simulink model "test_YAN_fusion"  (R2020b)
settings: Solver=ode1  StartTime=t0  StopTime=tf  FixedStep=0.004  RelTol=1e-3  EnableMultiTasking=on
values from neighbouring files (symbols this model uses):
  IMU = IN_SENSOR.IMU1    [run_simulation.m]
undefined symbols (not defined in the file or in its folder): accel_x, accel_y, accel_z, airspeed, airspeed1, airspeed2, airspeed3, airspeed_calibrate, airspeed_indicate, airspeed_true, alt_baro, baro1, baro2, BESTPOS, delta_height, delta_lat, delta_lon, dynamic_pressure, EAS2TAS_Algo, flag, Flag, glv, gyro_x, gyro_y, gyro_z, hAcc, headAcc, height, IMU1, IMU1_Control, IMU2, IMU3, IMU4, laserDown1, laserDown2, Lat, Lon, mag1, mag2, mag_x, mag_y, mag_z, nChange, numSv, pDop, radar1, radarLongDown1, radarLongForward1, range, Range, sAcc, SNR, static_pressure, status, strength, temperature, time, ublox1, um482, vAcc ... (+3)
(part 2 of 3)

== system test_YAN_fusion/SOURCE lookup table/laserDown1 ==
  time : Inport
  1-D Lookup Table1 : Lookup_n-D  NumberOfTableDimensions=1  BreakpointsForDimension1=IN_SENSOR.laserDown1.time(1:end-20)  Table=IN_SENSOR.laserDown1.range(1:end-20)  InterpMethod=Flat  ExtrapMethod=Clip  InternalRulePriority=Speed  RndMeth=Simplest  InputSameDT=on
  1-D Lookup Table2 : Lookup_n-D  NumberOfTableDimensions=1  BreakpointsForDimension1=IN_SENSOR.laserDown1.time(1:end-20)  Table=IN_SENSOR.laserDown1.flag(1:end-20)  InterpMethod=Flat  ExtrapMethod=Clip  InternalRulePriority=Speed  RndMeth=Simplest  InputSameDT=on
  1-D Lookup Table3 : Lookup_n-D  NumberOfTableDimensions=1  BreakpointsForDimension1=IN_SENSOR.laserDown1.time(1:end-20)  Table=IN_SENSOR.laserDown1.strength(1:end-20)  InterpMethod=Flat  ExtrapMethod=Clip  InternalRulePriority=Speed  RndMeth=Simplest  InputSameDT=on
  1-D Lookup Table4 : Lookup_n-D  NumberOfTableDimensions=1  BreakpointsForDimension1=IN_SENSOR.laserDown1.time(1:end-20)  Table=IN_SENSOR.laserDown1.nChange(1:end-20)  InterpMethod=Flat  ExtrapMethod=Clip  InternalRulePriority=Speed  RndMeth=Simplest  InputSameDT=on
  1-D Lookup Table9 : Lookup_n-D  NumberOfTableDimensions=1  BreakpointsForDimension1=IN_SENSOR.laserDown1.time(1:end-20)  Table=IN_SENSOR.laserDown1.time(1:end-20)  InterpMethod=Flat  ExtrapMethod=Clip  InternalRulePriority=Speed  RndMeth=Simplest  InputSameDT=on
  Bus Assignment : BusAssignment  AssignedSignals=time,range,flag,strength,nChange
  Constant : Constant  Value=0  OutDataTypeStr=Bus: BUS_LASERR_DOWN
  Data Type Conversion{,1..4} (5 alike) : DataTypeConversion
  Gain{1..3,8} (4 alike) : Gain
  Outport : Outport
  wires:
  time/1 -> 1-D Lookup Table1/1, 1-D Lookup Table9/1, 1-D Lookup Table2/1, 1-D Lookup Table4/1, 1-D Lookup Table3/1
  1-D Lookup Table3/1 -> Data Type Conversion3/1
  Data Type Conversion3/1 -> Gain3/1
  Data Type Conversion2/1 -> Gain2/1
  1-D Lookup Table2/1 -> Data Type Conversion2/1
  1-D Lookup Table1/1 -> Data Type Conversion1/1
  Data Type Conversion1/1 -> Gain1/1
  Data Type Conversion/1 -> Gain8/1
  1-D Lookup Table9/1 -> Data Type Conversion/1
  Gain3/1 -> Bus Assignment/5  "strength"
  Gain2/1 -> Bus Assignment/4  "flag"
  Gain8/1 -> Bus Assignment/2  "time"
  Gain1/1 -> Bus Assignment/3  "range"
  Constant/1 -> Bus Assignment/1
  Bus Assignment/1 -> Outport/1
  1-D Lookup Table4/1 -> Data Type Conversion4/1
  Data Type Conversion4/1 -> Bus Assignment/6  "nChange"

== system test_YAN_fusion/SOURCE lookup table/laserDown2 ==
  time : Inport
  1-D Lookup Table1 : Lookup_n-D  NumberOfTableDimensions=1  BreakpointsForDimension1=IN_SENSOR.laserDown2.time(1:end-20)  Table=IN_SENSOR.laserDown2.range(1:end-20)  InterpMethod=Flat  ExtrapMethod=Clip  InternalRulePriority=Speed  RndMeth=Simplest  InputSameDT=on
  1-D Lookup Table2 : Lookup_n-D  NumberOfTableDimensions=1  BreakpointsForDimension1=IN_SENSOR.laserDown2.time(1:end-20)  Table=IN_SENSOR.laserDown2.flag(1:end-20)  InterpMethod=Flat  ExtrapMethod=Clip  InternalRulePriority=Speed  RndMeth=Simplest  InputSameDT=on
  1-D Lookup Table3 : Lookup_n-D  NumberOfTableDimensions=1  BreakpointsForDimension1=IN_SENSOR.laserDown2.time(1:end-20)  Table=IN_SENSOR.laserDown2.strength(1:end-20)  InterpMethod=Flat  ExtrapMethod=Clip  InternalRulePriority=Speed  RndMeth=Simplest  InputSameDT=on
  1-D Lookup Table4 : Lookup_n-D  NumberOfTableDimensions=1  BreakpointsForDimension1=IN_SENSOR.laserDown2.time(1:end-20)  Table=IN_SENSOR.laserDown2.nChange(1:end-20)  InterpMethod=Flat  ExtrapMethod=Clip  InternalRulePriority=Speed  RndMeth=Simplest  InputSameDT=on
  1-D Lookup Table9 : Lookup_n-D  NumberOfTableDimensions=1  BreakpointsForDimension1=IN_SENSOR.laserDown2.time(1:end-20)  Table=IN_SENSOR.laserDown2.time(1:end-20)  InterpMethod=Flat  ExtrapMethod=Clip  InternalRulePriority=Speed  RndMeth=Simplest  InputSameDT=on
  Bus Assignment : BusAssignment  AssignedSignals=time,range,flag,strength,nChange
  Constant : Constant  Value=0  OutDataTypeStr=Bus: BUS_LASERR_DOWN
  Data Type Conversion{,1..4} (5 alike) : DataTypeConversion
  Gain{1..3,8} (4 alike) : Gain
  Outport : Outport
  wires:
  time/1 -> 1-D Lookup Table1/1, 1-D Lookup Table9/1, 1-D Lookup Table2/1, 1-D Lookup Table4/1, 1-D Lookup Table3/1
  1-D Lookup Table3/1 -> Data Type Conversion3/1
  Data Type Conversion3/1 -> Gain3/1
  Data Type Conversion2/1 -> Gain2/1
  1-D Lookup Table2/1 -> Data Type Conversion2/1
  1-D Lookup Table1/1 -> Data Type Conversion1/1
  Data Type Conversion1/1 -> Gain1/1
  Data Type Conversion/1 -> Gain8/1
  1-D Lookup Table9/1 -> Data Type Conversion/1
  Gain3/1 -> Bus Assignment/5  "strength"
  Gain2/1 -> Bus Assignment/4  "flag"
  Gain8/1 -> Bus Assignment/2  "time"
  Gain1/1 -> Bus Assignment/3  "range"
  Constant/1 -> Bus Assignment/1
  Data Type Conversion4/1 -> Bus Assignment/6  "nChange"
  1-D Lookup Table4/1 -> Data Type Conversion4/1
  Bus Assignment/1 -> Outport/1

== system test_YAN_fusion/SOURCE lookup table/mag1 ==
  time : Inport
  1-D Lookup Table1 : Lookup_n-D  NumberOfTableDimensions=1  BreakpointsForDimension1=IN_SENSOR.mag1.time(1:end-20)  Table=IN_SENSOR.mag1.mag_x(1:end-20)  InterpMethod=Flat  ExtrapMethod=Clip  InternalRulePriority=Speed  RndMeth=Simplest  InputSameDT=on
  1-D Lookup Table2 : Lookup_n-D  NumberOfTableDimensions=1  BreakpointsForDimension1=IN_SENSOR.mag1.time(1:end-20)  Table=IN_SENSOR.mag1.mag_y(1:end-20)  InterpMethod=Flat  ExtrapMethod=Clip  InternalRulePriority=Speed  RndMeth=Simplest  InputSameDT=on
  1-D Lookup Table3 : Lookup_n-D  NumberOfTableDimensions=1  BreakpointsForDimension1=IN_SENSOR.mag1.time(1:end-20)  Table=IN_SENSOR.mag1.mag_z(1:end-20)  InterpMethod=Flat  ExtrapMethod=Clip  InternalRulePriority=Speed  RndMeth=Simplest  InputSameDT=on
  1-D Lookup Table4 : Lookup_n-D  NumberOfTableDimensions=1  BreakpointsForDimension1=IN_SENSOR.mag1.time(1:end-20)  Table=IN_SENSOR.mag1.nChange(1:end-20)  InterpMethod=Flat  ExtrapMethod=Clip  InternalRulePriority=Speed  RndMeth=Simplest  InputSameDT=on
  1-D Lookup Table9 : Lookup_n-D  NumberOfTableDimensions=1  BreakpointsForDimension1=IN_SENSOR.mag1.time(1:end-20)  Table=IN_SENSOR.mag1.time(1:end-20)  InterpMethod=Flat  ExtrapMethod=Clip  InternalRulePriority=Speed  RndMeth=Simplest  InputSameDT=on
  Bus Assignment : BusAssignment  AssignedSignals=time,mag_x,mag_y,mag_z,nChange
  Constant : Constant  Value=0  OutDataTypeStr=Bus: BUS_MAG
  Data Type Conversion{,1..4} (5 alike) : DataTypeConversion
  Gain{1..4} (4 alike) : Gain
  Outport : Outport
  wires:
  Gain3/1 -> Bus Assignment/2  "time"
  Gain1/1 -> Bus Assignment/3  "mag_x"
  Gain4/1 -> Bus Assignment/5  "mag_z"
  Gain2/1 -> Bus Assignment/4  "mag_y"
  Data Type Conversion/1 -> Gain3/1
  1-D Lookup Table9/1 -> Data Type Conversion/1
  1-D Lookup Table1/1 -> Data Type Conversion1/1
  Data Type Conversion1/1 -> Gain1/1
  Data Type Conversion2/1 -> Gain2/1
  1-D Lookup Table2/1 -> Data Type Conversion2/1
  1-D Lookup Table3/1 -> Data Type Conversion3/1
  Data Type Conversion3/1 -> Gain4/1
  time/1 -> 1-D Lookup Table4/1, 1-D Lookup Table3/1, 1-D Lookup Table2/1, 1-D Lookup Table1/1, 1-D Lookup Table9/1
  Constant/1 -> Bus Assignment/1
  Bus Assignment/1 -> Outport/1
  1-D Lookup Table4/1 -> Data Type Conversion4/1
  Data Type Conversion4/1 -> Bus Assignment/6  "nChange"

== system test_YAN_fusion/SOURCE lookup table/mag2 ==
  time : Inport
  1-D Lookup Table1 : Lookup_n-D  NumberOfTableDimensions=1  BreakpointsForDimension1=IN_SENSOR.mag2.time(1:end-20)  Table=IN_SENSOR.mag2.mag_x(1:end-20)  InterpMethod=Flat  ExtrapMethod=Clip  InternalRulePriority=Speed  RndMeth=Simplest  InputSameDT=on
  1-D Lookup Table2 : Lookup_n-D  NumberOfTableDimensions=1  BreakpointsForDimension1=IN_SENSOR.mag2.time(1:end-20)  Table=IN_SENSOR.mag2.mag_y(1:end-20)  InterpMethod=Flat  ExtrapMethod=Clip  InternalRulePriority=Speed  RndMeth=Simplest  InputSameDT=on
  1-D Lookup Table3 : Lookup_n-D  NumberOfTableDimensions=1  BreakpointsForDimension1=IN_SENSOR.mag2.time(1:end-20)  Table=IN_SENSOR.mag2.mag_z(1:end-20)  InterpMethod=Flat  ExtrapMethod=Clip  InternalRulePriority=Speed  RndMeth=Simplest  InputSameDT=on
  1-D Lookup Table4 : Lookup_n-D  NumberOfTableDimensions=1  BreakpointsForDimension1=IN_SENSOR.mag2.time(1:end-20)  Table=IN_SENSOR.mag2.nChange(1:end-20)  InterpMethod=Flat  ExtrapMethod=Clip  InternalRulePriority=Speed  RndMeth=Simplest  InputSameDT=on
  1-D Lookup Table9 : Lookup_n-D  NumberOfTableDimensions=1  BreakpointsForDimension1=IN_SENSOR.mag2.time(1:end-20)  Table=IN_SENSOR.mag2.time(1:end-20)  InterpMethod=Flat  ExtrapMethod=Clip  InternalRulePriority=Speed  RndMeth=Simplest  InputSameDT=on
  Bus Assignment : BusAssignment  AssignedSignals=time,mag_x,mag_y,mag_z,nChange
  Constant : Constant  Value=0  OutDataTypeStr=Bus: BUS_MAG
  Data Type Conversion{,1..4} (5 alike) : DataTypeConversion
  Gain{1..4} (4 alike) : Gain
  Outport : Outport
  wires:
  Data Type Conversion4/1 -> Bus Assignment/6  "nChange"
  1-D Lookup Table4/1 -> Data Type Conversion4/1
  Bus Assignment/1 -> Outport/1
  Constant/1 -> Bus Assignment/1
  time/1 -> 1-D Lookup Table9/1, 1-D Lookup Table1/1, 1-D Lookup Table2/1, 1-D Lookup Table3/1, 1-D Lookup Table4/1
  Data Type Conversion3/1 -> Gain4/1
  1-D Lookup Table3/1 -> Data Type Conversion3/1
  1-D Lookup Table2/1 -> Data Type Conversion2/1
  Data Type Conversion2/1 -> Gain2/1
  Data Type Conversion1/1 -> Gain1/1
  1-D Lookup Table1/1 -> Data Type Conversion1/1
  1-D Lookup Table9/1 -> Data Type Conversion/1
  Data Type Conversion/1 -> Gain3/1
  Gain2/1 -> Bus Assignment/4  "mag_y"
  Gain4/1 -> Bus Assignment/5  "mag_z"
  Gain1/1 -> Bus Assignment/3  "mag_x"
  Gain3/1 -> Bus Assignment/2  "time"

== system test_YAN_fusion/SOURCE lookup table/radar1 ==
  time : Inport
  1-D Lookup Table1 : Lookup_n-D  NumberOfTableDimensions=1  BreakpointsForDimension1=IN_SENSOR.radar1.time(1:end-20)  Table=IN_SENSOR.radar1.SNR(1:end-20)  InterpMethod=Flat  ExtrapMethod=Clip  InternalRulePriority=Speed  RndMeth=Simplest  InputSameDT=on
  1-D Lookup Table2 : Lookup_n-D  NumberOfTableDimensions=1  BreakpointsForDimension1=IN_SENSOR.radar1.time(1:end-20)  Table=IN_SENSOR.radar1.Flag(1:end-20)  InterpMethod=Flat  ExtrapMethod=Clip  InternalRulePriority=Speed  RndMeth=Simplest  InputSameDT=on
  1-D Lookup Table3 : Lookup_n-D  NumberOfTableDimensions=1  BreakpointsForDimension1=IN_SENSOR.radar1.time(1:end-20)  Table=IN_SENSOR.radar1.Range(1:end-20)  InterpMethod=Flat  ExtrapMethod=Clip  InternalRulePriority=Speed  RndMeth=Simplest  InputSameDT=on
  1-D Lookup Table4 : Lookup_n-D  NumberOfTableDimensions=1  BreakpointsForDimension1=IN_SENSOR.radar1.time(1:end-20)  Table=IN_SENSOR.radar1.nChange(1:end-20)  InterpMethod=Flat  ExtrapMethod=Clip  InternalRulePriority=Speed  RndMeth=Simplest  InputSameDT=on
  1-D Lookup Table9 : Lookup_n-D  NumberOfTableDimensions=1  BreakpointsForDimension1=IN_SENSOR.radar1.time(1:end-20)  Table=IN_SENSOR.radar1.time(1:end-20)  InterpMethod=Flat  ExtrapMethod=Clip  InternalRulePriority=Speed  RndMeth=Simplest  InputSameDT=on
  Bus Assignment : BusAssignment  AssignedSignals=time,SNR,Flag,Range,nChange
  Constant : Constant  Value=0  OutDataTypeStr=Bus: BUS_RADAR
  Data Type Conversion{,1..4} (5 alike) : DataTypeConversion
  Gain{1..4} (4 alike) : Gain
  Outport : Outport
  wires:
  Gain3/1 -> Bus Assignment/2  "time"
  Gain1/1 -> Bus Assignment/3  "SNR"
  Gain4/1 -> Bus Assignment/5  "Range"
  Gain2/1 -> Bus Assignment/4  "Flag"
  1-D Lookup Table9/1 -> Data Type Conversion/1
  Data Type Conversion/1 -> Gain3/1
  Data Type Conversion1/1 -> Gain1/1
  1-D Lookup Table1/1 -> Data Type Conversion1/1
  1-D Lookup Table2/1 -> Data Type Conversion2/1
  Data Type Conversion2/1 -> Gain2/1
  Data Type Conversion3/1 -> Gain4/1
  1-D Lookup Table3/1 -> Data Type Conversion3/1
  time/1 -> 1-D Lookup Table4/1, 1-D Lookup Table3/1, 1-D Lookup Table2/1, 1-D Lookup Table1/1, 1-D Lookup Table9/1
  Constant/1 -> Bus Assignment/1
  Bus Assignment/1 -> Outport/1
  1-D Lookup Table4/1 -> Data Type Conversion4/1
  Data Type Conversion4/1 -> Bus Assignment/6  "nChange"

== system test_YAN_fusion/SOURCE lookup table/radarLongDown1 ==
  time : Inport
  1-D Lookup Table1 : Lookup_n-D  NumberOfTableDimensions=1  BreakpointsForDimension1=IN_SENSOR.radarLongDown1.time(1:end-20)  Table=IN_SENSOR.radarLongDown1.range(1:end-20)  InterpMethod=Flat  ExtrapMethod=Clip  InternalRulePriority=Speed  RndMeth=Simplest  InputSameDT=on
  1-D Lookup Table2 : Lookup_n-D  NumberOfTableDimensions=1  BreakpointsForDimension1=IN_SENSOR.radarLongDown1.time(1:end-20)  Table=IN_SENSOR.radarLongDown1.flag(1:end-20)  InterpMethod=Flat  ExtrapMethod=Clip  InternalRulePriority=Speed  RndMeth=Simplest  InputSameDT=on
  1-D Lookup Table3 : Lookup_n-D  NumberOfTableDimensions=1  BreakpointsForDimension1=IN_SENSOR.radarLongDown1.time(1:end-20)  Table=IN_SENSOR.radarLongDown1.strength(1:end-20)  InterpMethod=Flat  ExtrapMethod=Clip  InternalRulePriority=Speed  RndMeth=Simplest  InputSameDT=on
  1-D Lookup Table4 : Lookup_n-D  NumberOfTableDimensions=1  BreakpointsForDimension1=IN_SENSOR.radarLongDown1.time(1:end-20)  Table=IN_SENSOR.radarLongDown1.nChange(1:end-20)  InterpMethod=Flat  ExtrapMethod=Clip  InternalRulePriority=Speed  RndMeth=Simplest  InputSameDT=on
  1-D Lookup Table9 : Lookup_n-D  NumberOfTableDimensions=1  BreakpointsForDimension1=IN_SENSOR.radarLongDown1.time(1:end-20)  Table=IN_SENSOR.radarLongDown1.time(1:end-20)  InterpMethod=Flat  ExtrapMethod=Clip  InternalRulePriority=Speed  RndMeth=Simplest  InputSameDT=on
  Bus Assignment : BusAssignment  AssignedSignals=time,range,flag,strength,nChange
  Constant : Constant  Value=0  OutDataTypeStr=Bus: BUS_RADAR_LONG
  Data Type Conversion{,1..4} (5 alike) : DataTypeConversion
  Gain{1..3,8} (4 alike) : Gain
  Outport : Outport
  wires:
  Gain1/1 -> Bus Assignment/3  "range"
  Gain8/1 -> Bus Assignment/2  "time"
  Gain2/1 -> Bus Assignment/4  "flag"
  Gain3/1 -> Bus Assignment/5  "strength"
  1-D Lookup Table9/1 -> Data Type Conversion/1
  Data Type Conversion/1 -> Gain8/1
  Data Type Conversion1/1 -> Gain1/1
  1-D Lookup Table1/1 -> Data Type Conversion1/1
  1-D Lookup Table2/1 -> Data Type Conversion2/1
  Data Type Conversion2/1 -> Gain2/1
  Data Type Conversion3/1 -> Gain3/1
  1-D Lookup Table3/1 -> Data Type Conversion3/1
  time/1 -> 1-D Lookup Table4/1, 1-D Lookup Table3/1, 1-D Lookup Table9/1, 1-D Lookup Table1/1, 1-D Lookup Table2/1
  Constant/1 -> Bus Assignment/1
  Data Type Conversion4/1 -> Bus Assignment/6  "nChange"
  1-D Lookup Table4/1 -> Data Type Conversion4/1
  Bus Assignment/1 -> Outport/1

== system test_YAN_fusion/SOURCE lookup table/radarLongForward1 ==
  time : Inport
  1-D Lookup Table1 : Lookup_n-D  NumberOfTableDimensions=1  BreakpointsForDimension1=IN_SENSOR.radarLongForward1.time(1:end-20)  Table=IN_SENSOR.radarLongForward1.range(1:end-20)  InterpMethod=Flat  ExtrapMethod=Clip  InternalRulePriority=Speed  RndMeth=Simplest  InputSameDT=on
  1-D Lookup Table2 : Lookup_n-D  NumberOfTableDimensions=1  BreakpointsForDimension1=IN_SENSOR.radarLongForward1.time(1:end-20)  Table=IN_SENSOR.radarLongForward1.flag(1:end-20)  InterpMethod=Flat  ExtrapMethod=Clip  InternalRulePriority=Speed  RndMeth=Simplest  InputSameDT=on
  1-D Lookup Table3 : Lookup_n-D  NumberOfTableDimensions=1  BreakpointsForDimension1=IN_SENSOR.radarLongForward1.time(1:end-20)  Table=IN_SENSOR.radarLongForward1.strength(1:end-20)  InterpMethod=Flat  ExtrapMethod=Clip  InternalRulePriority=Speed  RndMeth=Simplest  InputSameDT=on
  1-D Lookup Table4 : Lookup_n-D  NumberOfTableDimensions=1  BreakpointsForDimension1=IN_SENSOR.radarLongForward1.time(1:end-20)  Table=IN_SENSOR.radarLongForward1.nChange(1:end-20)  InterpMethod=Flat  ExtrapMethod=Clip  InternalRulePriority=Speed  RndMeth=Simplest  InputSameDT=on
  1-D Lookup Table9 : Lookup_n-D  NumberOfTableDimensions=1  BreakpointsForDimension1=IN_SENSOR.radarLongForward1.time(1:end-20)  Table=IN_SENSOR.radarLongForward1.time(1:end-20)  InterpMethod=Flat  ExtrapMethod=Clip  InternalRulePriority=Speed  RndMeth=Simplest  InputSameDT=on
  Bus Assignment : BusAssignment  AssignedSignals=time,range,flag,strength,nChange
  Constant : Constant  Value=0  OutDataTypeStr=Bus: BUS_RADAR_LONG
  Data Type Conversion{,1..4} (5 alike) : DataTypeConversion
  Gain{1..3,8} (4 alike) : Gain
  Outport : Outport
  wires:
  time/1 -> 1-D Lookup Table1/1, 1-D Lookup Table9/1, 1-D Lookup Table2/1, 1-D Lookup Table4/1, 1-D Lookup Table3/1
  1-D Lookup Table3/1 -> Data Type Conversion3/1
  Data Type Conversion3/1 -> Gain3/1
  Data Type Conversion2/1 -> Gain2/1
  1-D Lookup Table2/1 -> Data Type Conversion2/1
  1-D Lookup Table1/1 -> Data Type Conversion1/1
  Data Type Conversion1/1 -> Gain1/1
  Data Type Conversion/1 -> Gain8/1
  1-D Lookup Table9/1 -> Data Type Conversion/1
  Gain3/1 -> Bus Assignment/5  "strength"
  Gain2/1 -> Bus Assignment/4  "flag"
  Gain8/1 -> Bus Assignment/2  "time"
  Gain1/1 -> Bus Assignment/3  "range"
  Constant/1 -> Bus Assignment/1
  Bus Assignment/1 -> Outport/1
  1-D Lookup Table4/1 -> Data Type Conversion4/1
  Data Type Conversion4/1 -> Bus Assignment/6  "nChange"

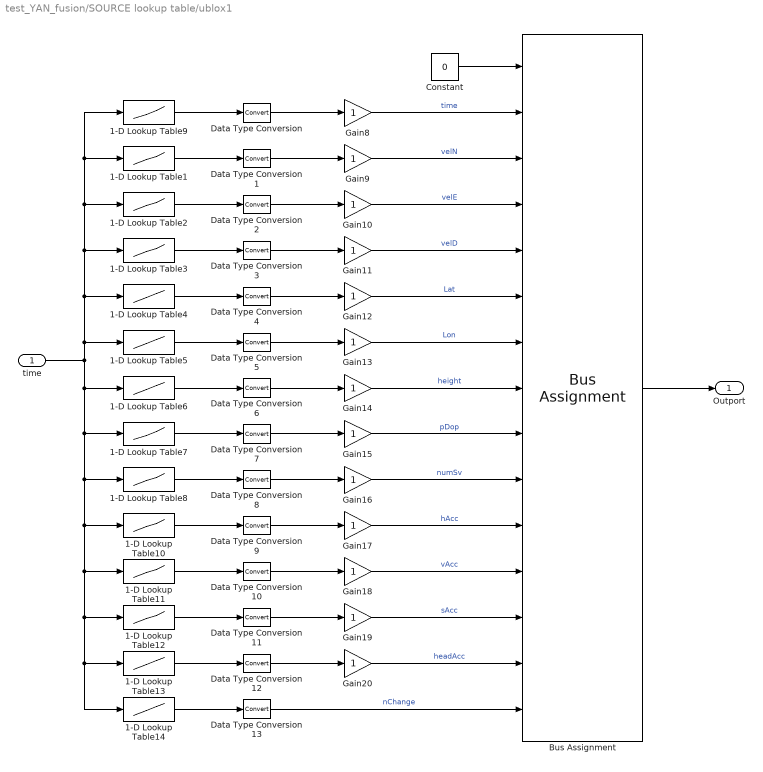
== system test_YAN_fusion/SOURCE lookup table/ublox1 ==
  time : Inport
  1-D Lookup Table1 : Lookup_n-D  NumberOfTableDimensions=1  BreakpointsForDimension1=IN_SENSOR.ublox1.time(1:end-20)  Table=IN_SENSOR.ublox1.velN(1:end-20)  InterpMethod=Flat  ExtrapMethod=Clip  InternalRulePriority=Speed  RndMeth=Simplest  InputSameDT=on
  1-D Lookup Table10 : Lookup_n-D  NumberOfTableDimensions=1  BreakpointsForDimension1=IN_SENSOR.ublox1.time(1:end-20)  Table=IN_SENSOR.ublox1.hAcc(1:end-20)  InterpMethod=Flat  ExtrapMethod=Clip  InternalRulePriority=Speed  RndMeth=Simplest  InputSameDT=on
  1-D Lookup Table11 : Lookup_n-D  NumberOfTableDimensions=1  BreakpointsForDimension1=IN_SENSOR.ublox1.time(1:end-20)  Table=IN_SENSOR.ublox1.vAcc(1:end-20)  InterpMethod=Flat  ExtrapMethod=Clip  InternalRulePriority=Speed  RndMeth=Simplest  InputSameDT=on
  1-D Lookup Table12 : Lookup_n-D  NumberOfTableDimensions=1  BreakpointsForDimension1=IN_SENSOR.ublox1.time(1:end-20)  Table=IN_SENSOR.ublox1.sAcc(1:end-20)  InterpMethod=Flat  ExtrapMethod=Clip  InternalRulePriority=Speed  RndMeth=Simplest  InputSameDT=on
  1-D Lookup Table13 : Lookup_n-D  NumberOfTableDimensions=1  BreakpointsForDimension1=IN_SENSOR.ublox1.time(1:end-20)  Table=IN_SENSOR.ublox1.headAcc(1:end-20)  InterpMethod=Flat  ExtrapMethod=Clip  InternalRulePriority=Speed  RndMeth=Simplest  InputSameDT=on
  1-D Lookup Table14 : Lookup_n-D  NumberOfTableDimensions=1  BreakpointsForDimension1=IN_SENSOR.ublox1.time(1:end-20)  Table=IN_SENSOR.ublox1.nChange(1:end-20)  InterpMethod=Flat  ExtrapMethod=Clip  InternalRulePriority=Speed  RndMeth=Simplest  InputSameDT=on
  1-D Lookup Table2 : Lookup_n-D  NumberOfTableDimensions=1  BreakpointsForDimension1=IN_SENSOR.ublox1.time(1:end-20)  Table=IN_SENSOR.ublox1.velE(1:end-20)  InterpMethod=Flat  ExtrapMethod=Clip  InternalRulePriority=Speed  RndMeth=Simplest  InputSameDT=on
  1-D Lookup Table3 : Lookup_n-D  NumberOfTableDimensions=1  BreakpointsForDimension1=IN_SENSOR.ublox1.time(1:end-20)  Table=IN_SENSOR.ublox1.velD(1:end-20)  InterpMethod=Flat  ExtrapMethod=Clip  InternalRulePriority=Speed  RndMeth=Simplest  InputSameDT=on
  1-D Lookup Table4 : Lookup_n-D  NumberOfTableDimensions=1  BreakpointsForDimension1=IN_SENSOR.ublox1.time(1:end-20)  Table=IN_SENSOR.ublox1.Lat(1:end-20)  InterpMethod=Flat  ExtrapMethod=Clip  InternalRulePriority=Speed  RndMeth=Simplest  InputSameDT=on
  1-D Lookup Table5 : Lookup_n-D  NumberOfTableDimensions=1  BreakpointsForDimension1=IN_SENSOR.ublox1.time(1:end-20)  Table=IN_SENSOR.ublox1.Lon(1:end-20)  InterpMethod=Flat  ExtrapMethod=Clip  InternalRulePriority=Speed  RndMeth=Simplest  InputSameDT=on
  1-D Lookup Table6 : Lookup_n-D  NumberOfTableDimensions=1  BreakpointsForDimension1=IN_SENSOR.ublox1.time(1:end-20)  Table=IN_SENSOR.ublox1.height(1:end-20)  InterpMethod=Flat  ExtrapMethod=Clip  InternalRulePriority=Speed  RndMeth=Simplest  InputSameDT=on
  1-D Lookup Table7 : Lookup_n-D  NumberOfTableDimensions=1  BreakpointsForDimension1=IN_SENSOR.ublox1.time(1:end-20)  Table=IN_SENSOR.ublox1.pDop(1:end-20)  InterpMethod=Flat  ExtrapMethod=Clip  InternalRulePriority=Speed  RndMeth=Simplest  InputSameDT=on
  1-D Lookup Table8 : Lookup_n-D  NumberOfTableDimensions=1  BreakpointsForDimension1=IN_SENSOR.ublox1.time(1:end-20)  Table=IN_SENSOR.ublox1.numSv(1:end-20)  InterpMethod=Flat  ExtrapMethod=Clip  InternalRulePriority=Speed  RndMeth=Simplest  InputSameDT=on
  1-D Lookup Table9 : Lookup_n-D  NumberOfTableDimensions=1  BreakpointsForDimension1=IN_SENSOR.ublox1.time(1:end-20)  Table=IN_SENSOR.ublox1.time(1:end-20)  InterpMethod=Flat  ExtrapMethod=Clip  InternalRulePriority=Speed  RndMeth=Simplest  InputSameDT=on
  Bus Assignment : BusAssignment  AssignedSignals=time,velN,velE,velD,Lat,Lon,height,pDop,numSv,hAcc,vAcc,sAcc,headAcc,nChange
  Constant : Constant  Value=0  OutDataTypeStr=Bus: BUS_UBLOX
  Data Type Conversion{,1..13} (14 alike) : DataTypeConversion
  Gain{8..20} (13 alike) : Gain
  Outport : Outport
  wires:
  Gain16/1 -> Bus Assignment/10  "numSv"
  Gain15/1 -> Bus Assignment/9  "pDop"
  Gain14/1 -> Bus Assignment/8  "height"
  Gain12/1 -> Bus Assignment/6  "Lat"
  Gain8/1 -> Bus Assignment/2  "time"
  Gain13/1 -> Bus Assignment/7  "Lon"
  Gain9/1 -> Bus Assignment/3  "velN"
  Gain10/1 -> Bus Assignment/4  "velE"
  Gain11/1 -> Bus Assignment/5  "velD"
  Gain17/1 -> Bus Assignment/11  "hAcc"
  Gain18/1 -> Bus Assignment/12  "vAcc"
  Gain19/1 -> Bus Assignment/13  "sAcc"
  Gain20/1 -> Bus Assignment/14  "headAcc"
  Data Type Conversion/1 -> Gain8/1
  1-D Lookup Table9/1 -> Data Type Conversion/1
  1-D Lookup Table1/1 -> Data Type Conversion1/1
  Data Type Conversion1/1 -> Gain9/1
  Data Type Conversion2/1 -> Gain10/1
  1-D Lookup Table2/1 -> Data Type Conversion2/1
  1-D Lookup Table3/1 -> Data Type Conversion3/1
  Data Type Conversion3/1 -> Gain11/1
  Data Type Conversion4/1 -> Gain12/1
  1-D Lookup Table4/1 -> Data Type Conversion4/1
  1-D Lookup Table5/1 -> Data Type Conversion5/1
  Data Type Conversion5/1 -> Gain13/1
  Data Type Conversion6/1 -> Gain14/1
  1-D Lookup Table6/1 -> Data Type Conversion6/1
  1-D Lookup Table7/1 -> Data Type Conversion7/1
  Data Type Conversion7/1 -> Gain15/1
  Data Type Conversion8/1 -> Gain16/1
  1-D Lookup Table8/1 -> Data Type Conversion8/1
  1-D Lookup Table10/1 -> Data Type Conversion9/1
  Data Type Conversion9/1 -> Gain17/1
  Data Type Conversion10/1 -> Gain18/1
  1-D Lookup Table11/1 -> Data Type Conversion10/1
  1-D Lookup Table12/1 -> Data Type Conversion11/1
  Data Type Conversion11/1 -> Gain19/1
  Data Type Conversion12/1 -> Gain20/1
  1-D Lookup Table13/1 -> Data Type Conversion12/1
  time/1 -> 1-D Lookup Table14/1, 1-D Lookup Table13/1, 1-D Lookup Table12/1, 1-D Lookup Table11/1, 1-D Lookup Table10/1, 1-D Lookup Table8/1, 1-D Lookup Table7/1, 1-D Lookup Table6/1, 1-D Lookup Table2/1, 1-D Lookup Table9/1, 1-D Lookup Table1/1, 1-D Lookup Table3/1, 1-D Lookup Table4/1, 1-D Lookup Table5/1
  Constant/1 -> Bus Assignment/1
  Bus Assignment/1 -> Outport/1
  1-D Lookup Table14/1 -> Data Type Conversion13/1
  Data Type Conversion13/1 -> Bus Assignment/15  "nChange"

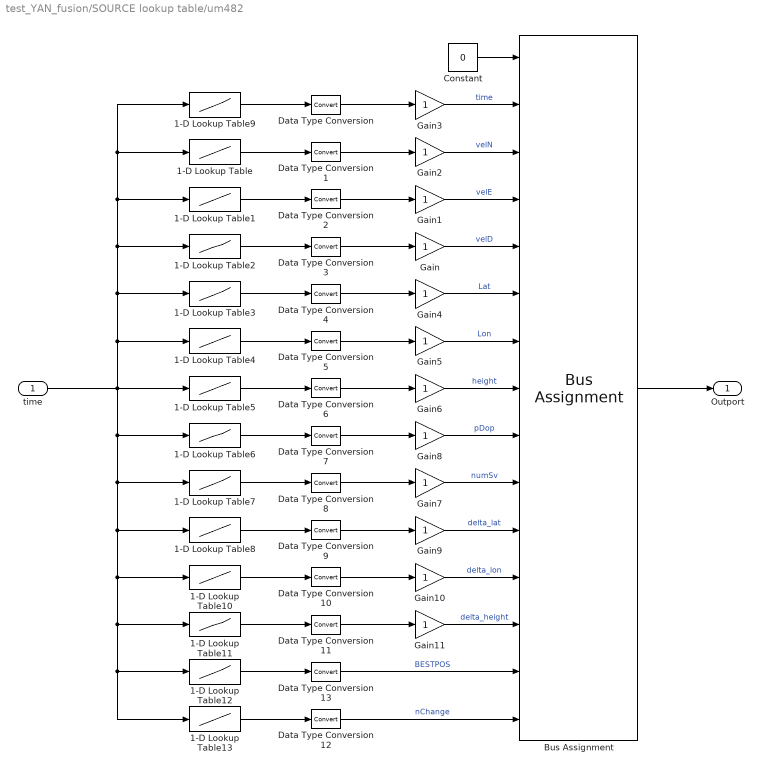
== system test_YAN_fusion/SOURCE lookup table/um482 ==
  time : Inport
  1-D Lookup Table : Lookup_n-D  NumberOfTableDimensions=1  BreakpointsForDimension1=IN_SENSOR.um482.time(1:end-20)  Table=IN_SENSOR.um482.velN(1:end-20)  InterpMethod=Flat  ExtrapMethod=Clip  InternalRulePriority=Speed  RndMeth=Simplest  InputSameDT=on
  1-D Lookup Table1 : Lookup_n-D  NumberOfTableDimensions=1  BreakpointsForDimension1=IN_SENSOR.um482.time(1:end-20)  Table=IN_SENSOR.um482.velE(1:end-20)  InterpMethod=Flat  ExtrapMethod=Clip  InternalRulePriority=Speed  RndMeth=Simplest  InputSameDT=on
  1-D Lookup Table10 : Lookup_n-D  NumberOfTableDimensions=1  BreakpointsForDimension1=IN_SENSOR.um482.time(1:end-20)  Table=IN_SENSOR.um482.delta_lon(1:end-20)  InterpMethod=Flat  ExtrapMethod=Clip  InternalRulePriority=Speed  RndMeth=Simplest  InputSameDT=on
  1-D Lookup Table11 : Lookup_n-D  NumberOfTableDimensions=1  BreakpointsForDimension1=IN_SENSOR.um482.time(1:end-20)  Table=IN_SENSOR.um482.delta_height(1:end-20)  InterpMethod=Flat  ExtrapMethod=Clip  InternalRulePriority=Speed  RndMeth=Simplest  InputSameDT=on
  1-D Lookup Table12 : Lookup_n-D  NumberOfTableDimensions=1  BreakpointsForDimension1=IN_SENSOR.um482.time(1:end-20)  Table=IN_SENSOR.um482.BESTPOS(1:end-20)  InterpMethod=Flat  ExtrapMethod=Clip  InternalRulePriority=Speed  RndMeth=Simplest  InputSameDT=on
  1-D Lookup Table13 : Lookup_n-D  NumberOfTableDimensions=1  BreakpointsForDimension1=IN_SENSOR.um482.time(1:end-20)  Table=IN_SENSOR.um482.nChange(1:end-20)  InterpMethod=Flat  ExtrapMethod=Clip  InternalRulePriority=Speed  RndMeth=Simplest  InputSameDT=on
  1-D Lookup Table2 : Lookup_n-D  NumberOfTableDimensions=1  BreakpointsForDimension1=IN_SENSOR.um482.time(1:end-20)  Table=IN_SENSOR.um482.velD(1:end-20)  InterpMethod=Flat  ExtrapMethod=Clip  InternalRulePriority=Speed  RndMeth=Simplest  InputSameDT=on
  1-D Lookup Table3 : Lookup_n-D  NumberOfTableDimensions=1  BreakpointsForDimension1=IN_SENSOR.um482.time(1:end-20)  Table=IN_SENSOR.um482.Lat(1:end-20)  InterpMethod=Flat  ExtrapMethod=Clip  InternalRulePriority=Speed  RndMeth=Simplest  InputSameDT=on
  1-D Lookup Table4 : Lookup_n-D  NumberOfTableDimensions=1  BreakpointsForDimension1=IN_SENSOR.um482.time(1:end-20)  Table=IN_SENSOR.um482.Lon(1:end-20)  InterpMethod=Flat  ExtrapMethod=Clip  InternalRulePriority=Speed  RndMeth=Simplest  InputSameDT=on
  1-D Lookup Table5 : Lookup_n-D  NumberOfTableDimensions=1  BreakpointsForDimension1=IN_SENSOR.um482.time(1:end-20)  Table=IN_SENSOR.um482.height(1:end-20)  InterpMethod=Flat  ExtrapMethod=Clip  InternalRulePriority=Speed  RndMeth=Simplest  InputSameDT=on
  1-D Lookup Table6 : Lookup_n-D  NumberOfTableDimensions=1  BreakpointsForDimension1=IN_SENSOR.um482.time(1:end-20)  Table=IN_SENSOR.um482.pDop(1:end-20)  InterpMethod=Flat  ExtrapMethod=Clip  InternalRulePriority=Speed  RndMeth=Simplest  InputSameDT=on
  1-D Lookup Table7 : Lookup_n-D  NumberOfTableDimensions=1  BreakpointsForDimension1=IN_SENSOR.um482.time(1:end-20)  Table=IN_SENSOR.um482.numSv(1:end-20)  InterpMethod=Flat  ExtrapMethod=Clip  InternalRulePriority=Speed  RndMeth=Simplest  InputSameDT=on
  1-D Lookup Table8 : Lookup_n-D  NumberOfTableDimensions=1  BreakpointsForDimension1=IN_SENSOR.um482.time(1:end-20)  Table=IN_SENSOR.um482.delta_lat(1:end-20)  InterpMethod=Flat  ExtrapMethod=Clip  InternalRulePriority=Speed  RndMeth=Simplest  InputSameDT=on
  1-D Lookup Table9 : Lookup_n-D  NumberOfTableDimensions=1  BreakpointsForDimension1=IN_SENSOR.um482.time(1:end-20)  Table=IN_SENSOR.um482.time(1:end-20)  InterpMethod=Flat  ExtrapMethod=Clip  InternalRulePriority=Speed  RndMeth=Simplest  InputSameDT=on
  Bus Assignment : BusAssignment  AssignedSignals=time,velN,velE,velD,Lat,Lon,height,pDop,numSv,delta_lat,delta_lon,delta_height,BESTPOS,nChange
  Constant : Constant  Value=0  OutDataTypeStr=Bus: BUS_UM482
  Data Type Conversion{,1..13} (14 alike) : DataTypeConversion
  Gain{,1..11} (12 alike) : Gain
  Outport : Outport
  wires:
  Gain4/1 -> Bus Assignment/6  "Lat"
  Gain6/1 -> Bus Assignment/8  "height"
  Gain1/1 -> Bus Assignment/4  "velE"
  Gain7/1 -> Bus Assignment/10  "numSv"
  Gain/1 -> Bus Assignment/5  "velD"
  Gain3/1 -> Bus Assignment/2  "time"
  Gain2/1 -> Bus Assignment/3  "velN"
  Gain5/1 -> Bus Assignment/7  "Lon"
  Gain8/1 -> Bus Assignment/9  "pDop"
  Gain9/1 -> Bus Assignment/11  "delta_lat"
  Gain10/1 -> Bus Assignment/12  "delta_lon"
  Gain11/1 -> Bus Assignment/13  "delta_height"
  Data Type Conversion13/1 -> Bus Assignment/14  "BESTPOS"
  time/1 -> 1-D Lookup Table11/1, 1-D Lookup Table13/1, 1-D Lookup Table12/1, 1-D Lookup Table10/1, 1-D Lookup Table8/1, 1-D Lookup Table7/1, 1-D Lookup Table6/1, 1-D Lookup Table9/1, 1-D Lookup Table/1, 1-D Lookup Table1/1, 1-D Lookup Table2/1, 1-D Lookup Table3/1, 1-D Lookup Table4/1, 1-D Lookup Table5/1
  1-D Lookup Table9/1 -> Data Type Conversion/1
  Data Type Conversion/1 -> Gain3/1
  Data Type Conversion1/1 -> Gain2/1
  1-D Lookup Table/1 -> Data Type Conversion1/1
  1-D Lookup Table2/1 -> Data Type Conversion3/1
  Data Type Conversion3/1 -> Gain/1
  Data Type Conversion2/1 -> Gain1/1
  1-D Lookup Table1/1 -> Data Type Conversion2/1
  1-D Lookup Table5/1 -> Data Type Conversion6/1
  Data Type Conversion6/1 -> Gain6/1
  Data Type Conversion7/1 -> Gain8/1
  1-D Lookup Table6/1 -> Data Type Conversion7/1
  1-D Lookup Table4/1 -> Data Type Conversion5/1
  Data Type Conversion5/1 -> Gain5/1
  Data Type Conversion4/1 -> Gain4/1
  1-D Lookup Table3/1 -> Data Type Conversion4/1
  1-D Lookup Table8/1 -> Data Type Conversion9/1
  Data Type Conversion9/1 -> Gain9/1
  Data Type Conversion10/1 -> Gain10/1
  1-D Lookup Table10/1 -> Data Type Conversion10/1
  1-D Lookup Table12/1 -> Data Type Conversion13/1
  Data Type Conversion11/1 -> Gain11/1
  1-D Lookup Table11/1 -> Data Type Conversion11/1
  Data Type Conversion8/1 -> Gain7/1
  1-D Lookup Table7/1 -> Data Type Conversion8/1
  Constant/1 -> Bus Assignment/1
  Bus Assignment/1 -> Outport/1
  1-D Lookup Table13/1 -> Data Type Conversion12/1
  Data Type Conversion12/1 -> Bus Assignment/15  "nChange"
